simulink model "RC_CIRCUIT1"  (R2023a)
settings: Solver=VariableStepAuto  StartTime=0.0  StopTime=10.0  RelTol=1e-3
values from neighbouring files (symbols this model uses):
  C = 1*10^-6    (= 1e-06)    [RC_CIRCUIT.m]
  R = Resistor_values(i)    [RC_CIRCUIT.m]
settings Model: Creator=alaam  LastModifiedBy=alaam

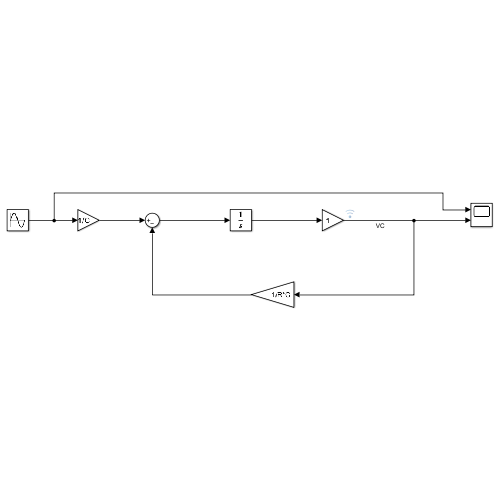
[thumbnail: Simulink's stored preview of the top-level diagram]
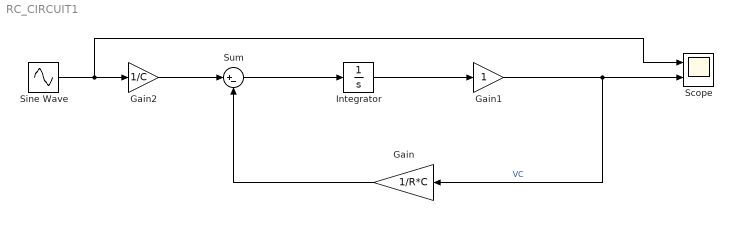
== system RC_CIRCUIT1 ==
  Gain : Gain  Gain=1/R*C
  Gain1 : Gain
  Gain2 : Gain  Gain=1/C
  Integrator : Integrator
  Scope : Scope  NumInputPorts=2
  Sine Wave : Sin  Amplitude=5  Phase=2*pi*1  SampleTime=0
  Sum : Sum  Inputs=|+-
  wires:
  Integrator/1 -> Gain1/1
  Sine Wave/1 -> Scope/1, Gain2/1
  Gain2/1 -> Sum/1
  Gain/1 -> Sum/2
  Gain1/1 -> Gain/1, Scope/2  "VC"
  Sum/1 -> Integrator/1
